simulink model "sampleModel106"  (R2022a)
settings: Solver=VariableStepAuto  StartTime=0.0  StopTime=10.0  RelTol=1e-3
undefined symbols (not defined in the file): DiscIntNeverNeededParam, magnitude, Newton, Raphson
libraries: simulink x379, slpidlib x89
(part 3 of 16)

== system sampleModel106/cfblk74/cfblk13/cfblk11 ==
  cfblk1 : Inport
  cfblk12 : Inport  Port=2
  cfblk10 : Subsystem
  cfblk11 : If  IfExpression=u1 >= 0  SampleTime=1
  cfblk14 : Subsystem  TreatAsAtomicUnit=on
  cfblk15 : Subsystem  TreatAsAtomicUnit=on
  cfblk{16..20} (5 alike) : Delay  SampleTime=1
  cfblk3 : slpidlib/PID Controller (2DOF)  Controller=PID  Form=Parallel  TimeDomain=Discrete-time  UseExternalTs=off  SampleTime=1  IntegratorMethod=Forward Euler  FilterMethod=Forward Euler  ControllerParametersSource=internal  P=1  I=1  UseKiTs=off  D=0  N=100  UseFilter=on  b=1  c=1  TunerSelectOption=Transfer Function Based (PID Tuner App)  InitialConditionSource=internal  InitialConditionForIntegrator=0  InitialConditionForFilter=0  DifferentiatorICPrevScaledInput=0  ExternalReset=none  TrackingMode=off  Kt=1  LimitOutput=off  SatLimitsSource=internal  UpperSaturationLimit=inf  LowerSaturationLimit=-inf  LinearizeAsGain=off  AntiWindupMode=none  Kb=1  POutMin=[]  POutMax=[]  IOutMin=[]  IOutMax=[]  DOutMin=[]  DOutMax=[]  NOutMin=[]  NOutMax=[]  bOutMin=[]  bOutMax=[]  cOutMin=[]  cOutMax=[]  SumOutMin=[]  SumOutMax=[]  SaturationOutMin=[]  SaturationOutMax=[]  PParamMin=[]  PParamMax=[]  IParamMin=[]  IParamMax=[]  DParamMin=[]  DParamMax=[]  NParamMin=[]  NParamMax=[]  bParamMin=[]  bParamMax=[]  cParamMin=[]  cParamMax=[]  KbParamMin=[]  KbParamMax=[]  KtParamMin=[]  KtParamMax=[]  KbOutMin=[]  KbOutMax=[]  KtOutMin=[]  KtOutMax=[]  IntegratorOutMin=[]  IntegratorOutMax=[]  FilterOutMin=[]  FilterOutMax=[]  SumI1OutMin=[]  SumI1OutMax=[]  SumI2OutMin=[]  SumI2OutMax=[]  SumI3OutMin=[]  SumI3OutMax=[]  SumI4OutMin=[]  SumI4OutMax=[]  SumDOutMin=[]  SumDOutMax=[]  Sum1OutMin=[]  Sum1OutMax=[]  Sum2OutMin=[]  Sum2OutMax=[]  Sum3OutMin=[]  Sum3OutMax=[]  DifferentiatorOutMin=[]  DifferentiatorOutMax=[]  FilterDiffOutCoefMin=[]  FilterDiffOutCoefMax=[]  ReciprocalOutMin=[]  ReciprocalOutMax=[]  SumDenOutMin=[]  SumDenOutMax=[]  SumNumOutMin=[]  SumNumOutMax=[]  DivideOutMin=[]  DivideOutMax=[]  UdiffTsProdOutMin=[]  UdiffTsProdOutMax=[]  NTsProdOutMin=[]  NTsProdOutMax=[]  UintegralTsProdOutMin=[]  UintegralTsProdOutMax=[]  UngainTsProdOutMin=[]  UngainTsProdOutMax=[]  IntegratorContinuousStateAttributes=''  IntegratorStateMustResolveToSignalObject=off  IntegratorRTWStateStorageClass=Auto  FilterContinuousStateAttributes=''  FilterStateMustResolveToSignalObject=off  FilterRTWStateStorageClass=Auto  ParallelPVariant=InternalParameters  IdealPVariant=Disabled  IVariant=InternalParameters  DVariant=InternalParameters  bVariant=InternalParameters  cVariant=InternalParameters  IntegratorVariant=Discrete  SatVariant=Disabled  AWVariant=Passthrough  PCopyVariant=Disabled  TRVariant=Disabled  FdbkBlocksVariant=Forward  IdealPFdbkVariant=Disabled  SatFdbkVariant=Disabled  DerivativeFilterVariant=ForwardEulerFilter  NVariant=InternalParameters  NCopyVariant=Disabled  FilterICVariant=InternalICsFilter  IntegratorICVariant=InternalICs  ExternalResetVariant=Disabled  TRSumVariant=Passthrough  SumFdbkVariant=Disabled  SumVariant=Sum_PID  TsampFilterVariant=InternalTs  TsampNgainVariant=Passthrough  TsampIntegralVariant=Passthrough  ExternalSaturationOutDataTypeStr=Inherit: Same as second input
      settings: SourceProductBaseCode=SL
  cfblk4 : DiscreteFilter  SampleTime=1
  cfblk5 : Squeeze
  cfblk6 : Constant  Value=[-862764176.620188]  SampleTime=1
  cfblk7 : Subsystem
  cfblk8 : Subsystem
  cfblk9 : Subsystem
  cfblk2 : Outport
  cfblk13 : Outport  Port=2
  wires:
  cfblk4/1 -> cfblk5/1, cfblk3/2, cfblk15/4(cfblk9)
  cfblk9/1(cfblk2) -> cfblk4/1
  cfblk1/1 -> cfblk10/1(cfblk1), cfblk15/5(cfblk10), cfblk15/6(cfblk11)
  cfblk3/1 -> cfblk13/1
  cfblk10/1(cfblk2) -> cfblk2/1
  cfblk14/2(cfblk15) -> cfblk8/1(cfblk1)
  cfblk9/2(cfblk11) -> cfblk7/1(cfblk1)
  cfblk12/1 -> cfblk7/2(cfblk11)
  cfblk9/3(cfblk12) -> cfblk14/1(cfblk1), cfblk7/6(cfblk15)
  cfblk6/1 -> cfblk14/2(cfblk13)
  cfblk10/2(cfblk11) -> cfblk9/3(cfblk10)
  cfblk10/3(cfblk12) -> cfblk14/3(cfblk14)
  cfblk14/4(cfblk17) -> cfblk8/2(cfblk13), cfblk15/1(cfblk1)
  cfblk15/1(cfblk2) -> cfblk7/3(cfblk12)
  cfblk10/4(cfblk13) -> cfblk8/3(cfblk14)
  cfblk5/1 -> cfblk7/4(cfblk13), cfblk15/3(cfblk8)
  cfblk10/5(cfblk14) -> cfblk11/1
  cfblk8/1(cfblk2) -> cfblk7/5(cfblk14)
  cfblk8/2(cfblk15) -> cfblk3/1, cfblk19/1
  cfblk11/1 -> cfblk14/Action
  cfblk11/2 -> cfblk15/Action
  cfblk7/1(cfblk2) -> cfblk16/1
  cfblk16/1 -> cfblk10/2(cfblk9)
  cfblk7/2(cfblk16) -> cfblk17/1
  cfblk17/1 -> cfblk9/2(cfblk9)
  cfblk14/1(cfblk2) -> cfblk18/1
  cfblk18/1 -> cfblk9/1(cfblk1)
  cfblk19/1 -> cfblk15/2(cfblk7)
  cfblk14/3(cfblk16) -> cfblk20/1
  cfblk20/1 -> cfblk10/3(cfblk10)

== system sampleModel106/cfblk74/cfblk13/cfblk12 ==
  cfblk1 : Inport
  cfblk11 : Inport  Port=2
  cfblk12 : Inport  Port=3
  cfblk13 : Inport  Port=4
  cfblk10 : Subsystem
  cfblk3 : simulink/Discrete/Transfer Fcn First Order  PoleZ=0.95  ICPrevOutput=0.0  DoSatur=off
  cfblk4 : DiscreteTransferFcn  SampleTime=1
  cfblk5 : simulink/Discrete/Difference  ICPrevInput=0.0  OutMin=[]  OutMax=[]  OutDataTypeStr=Inherit: Inherit via back propagation  OutDataType=fixdt(1, 16)  OutScaling=2^-10  DoSatur=off
  cfblk6 : Math  Operator=mod
  cfblk7 : Product  Inputs=**
  cfblk8 : Constant  Value=[-371034601.961383]  SampleTime=1
  cfblk9 : Constant  Value=[478763481.548670]  SampleTime=1
  cfblk2 : Outport
  cfblk14 : Outport  Port=2
  wires:
  cfblk1/1 -> cfblk7/1
  cfblk13/1 -> cfblk4/1
  cfblk9/1 -> cfblk5/1
  cfblk10/1(cfblk2) -> cfblk6/1
  cfblk4/1 -> cfblk10/1(cfblk1)
  cfblk10/2(cfblk10) -> cfblk6/2
  cfblk3/1 -> cfblk7/2
  cfblk8/1 -> cfblk10/2(cfblk8)
  cfblk11/1 -> cfblk14/1
  cfblk6/1 -> cfblk2/1
  cfblk5/1 -> cfblk3/1
  cfblk12/1 -> cfblk10/3(cfblk9)

== system sampleModel106/cfblk74/cfblk13/cfblk13 ==
  cfblk1 : Inport
  cfblk13 : Inport  Port=2
  cfblk14 : Inport  Port=3
  cfblk10 : Subsystem
  cfblk11 : Subsystem
  cfblk12 : Subsystem
  cfblk15 : Delay  SampleTime=1
  cfblk16 : Delay  SampleTime=1
  cfblk3 : Delay  DelayLengthSource=Input port  SampleTime=1
      settings: InputPortMap=u0,p1
  cfblk4 : Product  Inputs=*
  cfblk5 : MinMax  Function=max  Inputs=3
  cfblk6 : Constant  Value=[-504496130.229108]  SampleTime=1
  cfblk7 : Constant  Value=[-450280739.885704]  SampleTime=1
  cfblk8 : Constant  Value=[-820475792.542349]  SampleTime=1
  cfblk9 : Subsystem
  cfblk2 : Outport
  wires:
  cfblk13/1 -> cfblk4/1
  cfblk14/1 -> cfblk12/1(cfblk1), cfblk10/5(cfblk15)
  cfblk11/1(cfblk2) -> cfblk10/1(cfblk1)
  cfblk4/1 -> cfblk11/1(cfblk1)
  cfblk5/1 -> cfblk3/1
  cfblk7/1 -> cfblk5/2
  cfblk9/1(cfblk2) -> cfblk5/3
  cfblk6/1 -> cfblk2/1
  cfblk8/1 -> cfblk10/2(cfblk12)
  cfblk12/1(cfblk2) -> cfblk3/2
  cfblk1/1 -> cfblk10/4(cfblk14)
  cfblk12/2(cfblk12) -> cfblk9/1(cfblk1)
  cfblk10/1(cfblk2) -> cfblk9/2(cfblk7)
  cfblk3/1 -> cfblk15/1
  cfblk15/1 -> cfblk5/1
  cfblk9/2(cfblk8) -> cfblk16/1
  cfblk16/1 -> cfblk10/3(cfblk13)

== system sampleModel106/cfblk74/cfblk9/cfblk10 ==
  cfblk1 : Inport
  cfblk7 : Inport  Port=2
  cfblk3 : DiscreteZeroPole  Poles=[0 0.5]  Gain=1
  cfblk4 : Reshape
  cfblk5 : Sum  Inputs=+
  cfblk6 : Constant  Value=[-238352155.093476]  SampleTime=1
  cfblk2 : Outport
  wires:
  cfblk6/1 -> cfblk3/1
  cfblk5/1 -> cfblk4/1
  cfblk4/1 -> cfblk2/1
  cfblk7/1 -> cfblk5/1

== system sampleModel106/cfblk74/cfblk9/cfblk11 ==
  cfblk1 : Inport
  cfblk10 : Inport  Port=2
  cfblk11 : Delay  SampleTime=1
  cfblk12 : Delay  SampleTime=1
  cfblk3 : slpidlib/PID Controller (2DOF)  Controller=PID  Form=Parallel  TimeDomain=Discrete-time  UseExternalTs=off  SampleTime=1  IntegratorMethod=Forward Euler  FilterMethod=Forward Euler  ControllerParametersSource=internal  P=1  I=1  UseKiTs=off  D=0  N=100  UseFilter=on  b=1  c=1  TunerSelectOption=Transfer Function Based (PID Tuner App)  InitialConditionSource=internal  InitialConditionForIntegrator=0  InitialConditionForFilter=0  DifferentiatorICPrevScaledInput=0  ExternalReset=none  TrackingMode=off  Kt=1  LimitOutput=off  SatLimitsSource=internal  UpperSaturationLimit=inf  LowerSaturationLimit=-inf  LinearizeAsGain=off  AntiWindupMode=none  Kb=1  POutMin=[]  POutMax=[]  IOutMin=[]  IOutMax=[]  DOutMin=[]  DOutMax=[]  NOutMin=[]  NOutMax=[]  bOutMin=[]  bOutMax=[]  cOutMin=[]  cOutMax=[]  SumOutMin=[]  SumOutMax=[]  SaturationOutMin=[]  SaturationOutMax=[]  PParamMin=[]  PParamMax=[]  IParamMin=[]  IParamMax=[]  DParamMin=[]  DParamMax=[]  NParamMin=[]  NParamMax=[]  bParamMin=[]  bParamMax=[]  cParamMin=[]  cParamMax=[]  KbParamMin=[]  KbParamMax=[]  KtParamMin=[]  KtParamMax=[]  KbOutMin=[]  KbOutMax=[]  KtOutMin=[]  KtOutMax=[]  IntegratorOutMin=[]  IntegratorOutMax=[]  FilterOutMin=[]  FilterOutMax=[]  SumI1OutMin=[]  SumI1OutMax=[]  SumI2OutMin=[]  SumI2OutMax=[]  SumI3OutMin=[]  SumI3OutMax=[]  SumI4OutMin=[]  SumI4OutMax=[]  SumDOutMin=[]  SumDOutMax=[]  Sum1OutMin=[]  Sum1OutMax=[]  Sum2OutMin=[]  Sum2OutMax=[]  Sum3OutMin=[]  Sum3OutMax=[]  DifferentiatorOutMin=[]  DifferentiatorOutMax=[]  FilterDiffOutCoefMin=[]  FilterDiffOutCoefMax=[]  ReciprocalOutMin=[]  ReciprocalOutMax=[]  SumDenOutMin=[]  SumDenOutMax=[]  SumNumOutMin=[]  SumNumOutMax=[]  DivideOutMin=[]  DivideOutMax=[]  UdiffTsProdOutMin=[]  UdiffTsProdOutMax=[]  NTsProdOutMin=[]  NTsProdOutMax=[]  UintegralTsProdOutMin=[]  UintegralTsProdOutMax=[]  UngainTsProdOutMin=[]  UngainTsProdOutMax=[]  IntegratorContinuousStateAttributes=''  IntegratorStateMustResolveToSignalObject=off  IntegratorRTWStateStorageClass=Auto  FilterContinuousStateAttributes=''  FilterStateMustResolveToSignalObject=off  FilterRTWStateStorageClass=Auto  ParallelPVariant=InternalParameters  IdealPVariant=Disabled  IVariant=InternalParameters  DVariant=InternalParameters  bVariant=InternalParameters  cVariant=InternalParameters  IntegratorVariant=Discrete  SatVariant=Disabled  AWVariant=Passthrough  PCopyVariant=Disabled  TRVariant=Disabled  FdbkBlocksVariant=Forward  IdealPFdbkVariant=Disabled  SatFdbkVariant=Disabled  DerivativeFilterVariant=ForwardEulerFilter  NVariant=InternalParameters  NCopyVariant=Disabled  FilterICVariant=InternalICsFilter  IntegratorICVariant=InternalICs  ExternalResetVariant=Disabled  TRSumVariant=Passthrough  SumFdbkVariant=Disabled  SumVariant=Sum_PID  TsampFilterVariant=InternalTs  TsampNgainVariant=Passthrough  TsampIntegralVariant=Passthrough  ExternalSaturationOutDataTypeStr=Inherit: Same as second input
      settings: SourceProductBaseCode=SL
  cfblk4 : DiscreteTransferFcn  SampleTime=1
  cfblk5 : DotProduct  OutDataTypeStr=Inherit: Inherit via internal rule
  cfblk6 : ComplexToMagnitudeAngle
  cfblk7 : Constant  Value=[-659082313.129839]  SampleTime=1
  cfblk8 : Subsystem
  cfblk9 : Subsystem
  cfblk2 : Outport
  wires:
  cfblk9/1(cfblk2) -> cfblk4/1
  cfblk10/1 -> cfblk9/1(cfblk1)
  cfblk3/1 -> cfblk6/1
  cfblk7/1 -> cfblk8/2(cfblk9)
  cfblk8/1(cfblk2) -> cfblk2/1
  cfblk6/1 -> cfblk8/3(cfblk10)
  cfblk1/1 -> cfblk3/2
  cfblk8/2(cfblk11) -> cfblk9/2(cfblk8)
  cfblk4/1 -> cfblk5/1
  cfblk6/2 -> cfblk5/2
  cfblk5/1 -> cfblk11/1
  cfblk11/1 -> cfblk8/1(cfblk1)
  cfblk9/2(cfblk9) -> cfblk12/1
  cfblk12/1 -> cfblk3/1

== system sampleModel106/cfblk74/cfblk9/cfblk12 ==
  cfblk1 : Inport
  cfblk10 : Subsystem
  cfblk11 : If  IfExpression=u1 >= 0  SampleTime=1
  cfblk13 : Subsystem  TreatAsAtomicUnit=on
  cfblk14 : Subsystem  TreatAsAtomicUnit=on
  cfblk{15..21} (7 alike) : Delay  SampleTime=1
  cfblk3 : UnaryMinus
  cfblk4 : Sum  Inputs=+-
  cfblk5 : Squeeze
  cfblk6 : Constant  Value=[744843425.057498]  SampleTime=1
  cfblk7 : Constant  Value=[784568269.900237]  SampleTime=1
  cfblk8 : Subsystem
  cfblk9 : Subsystem
  cfblk2 : Outport
  cfblk12 : Outport  Port=2
  wires:
  cfblk1/1 -> cfblk8/1(cfblk1), cfblk9/2(cfblk8)
  cfblk5/1 -> cfblk12/1, cfblk9/4(cfblk10), cfblk2/1
  cfblk9/1(cfblk2) -> cfblk14/2(cfblk9)
  cfblk6/1 -> cfblk13/1(cfblk1), cfblk4/1, cfblk4/2
  cfblk7/1 -> cfblk10/1(cfblk1), cfblk9/3(cfblk9)
  cfblk4/1 -> cfblk14/3(cfblk10)
  cfblk8/1(cfblk2) -> cfblk5/1
  cfblk14/1(cfblk2) -> cfblk10/3(cfblk7)
  cfblk10/1(cfblk2) -> cfblk15/1, cfblk20/1, cfblk21/1
  cfblk14/2(cfblk12) -> cfblk13/2(cfblk12)
  cfblk13/4(cfblk16) -> cfblk3/1
  cfblk11/1 -> cfblk13/Action
  cfblk11/2 -> cfblk14/Action
  cfblk15/1 -> cfblk14/4(cfblk11)
  cfblk13/1(cfblk2) -> cfblk16/1
  cfblk16/1 -> cfblk10/2(cfblk6)
  cfblk13/2(cfblk14) -> cfblk17/1
  cfblk17/1 -> cfblk8/2(cfblk7)
  cfblk13/3(cfblk15) -> cfblk18/1
  cfblk18/1 -> cfblk9/1(cfblk1)
  cfblk3/1 -> cfblk19/1
  cfblk19/1 -> cfblk14/1(cfblk1)
  cfblk20/1 -> cfblk11/1
  cfblk21/1 -> cfblk13/3(cfblk13)

== system sampleModel106/cfblk74/cfblk9/cfblk13 ==
  cfblk1 : Inport
  cfblk10 : Delay  SampleTime=1
  cfblk3 : Sum  Inputs=|++
  cfblk4 : Constant  Value=[-872842553.263368]  SampleTime=1
  cfblk5 : Subsystem
  cfblk6 : Subsystem
  cfblk7 : Subsystem
  cfblk8 : Delay  SampleTime=1
  cfblk9 : Delay  SampleTime=1
  cfblk2 : Outport
  wires:
  cfblk5/1(cfblk2) -> cfblk3/1
  cfblk3/1 -> cfblk7/1(cfblk1)
  cfblk1/1 -> cfblk6/1(cfblk1)
  cfblk4/1 -> cfblk3/2
  cfblk5/2(cfblk10) -> cfblk9/1, cfblk10/1
  cfblk6/1(cfblk2) -> cfblk5/2(cfblk9)
  cfblk7/2(cfblk13) -> cfblk2/1
  cfblk7/1(cfblk2) -> cfblk8/1
  cfblk8/1 -> cfblk5/1(cfblk1)
  cfblk9/1 -> cfblk6/2(cfblk7)
  cfblk10/1 -> cfblk6/3(cfblk8)

== system sampleModel106/cfblk74/cfblk9/cfblk14 ==
  cfblk1 : Inport
  cfblk7 : Inport  Port=2
  cfblk3 : DiscreteIntegrator  ICPrevOutput=DiscIntNeverNeededParam  ICPrevScaledInput=DiscIntNeverNeededParam
  cfblk4 : DiscreteTransferFcn  SampleTime=1
  cfblk5 : PermuteDimensions
  cfblk6 : ComplexToRealImag
  cfblk2 : Outport
  cfblk8 : Outport  Port=2
  cfblk9 : Outport  Port=3
  cfblk10 : Outport  Port=4
  wires:
  cfblk7/1 -> cfblk10/1, cfblk5/1
  cfblk6/1 -> cfblk9/1
  cfblk5/1 -> cfblk3/1
  cfblk6/2 -> cfblk4/1
  cfblk4/1 -> cfblk2/1
  cfblk1/1 -> cfblk8/1
  cfblk3/1 -> cfblk6/1

== system sampleModel106/cfblk74/cfblk9/cfblk15 ==
  cfblk1 : Inport
  cfblk12 : Inport  Port=2
  cfblk10 : Subsystem
  cfblk11 : Subsystem
  cfblk{3,13..16} (5 alike) : Delay  SampleTime=1
  cfblk4 : Sum  Inputs=--
  cfblk5 : Trigonometry
  cfblk6 : Reshape
  cfblk7 : Rounding
  cfblk8 : Constant  Value=[-157824095.994580]  SampleTime=1
  cfblk9 : Subsystem
  cfblk2 : Outport
  wires:
  cfblk5/1 -> cfblk3/1
  cfblk9/1(cfblk2) -> cfblk5/1
  cfblk3/1 -> cfblk7/1
  cfblk7/1 -> cfblk14/1, cfblk15/1
  cfblk8/1 -> cfblk2/1
  cfblk1/1 -> cfblk4/1
  cfblk4/1 -> cfblk11/2(cfblk13)
  cfblk12/1 -> cfblk10/1(cfblk1)
  cfblk6/1 -> cfblk10/2(cfblk11)
  cfblk10/1(cfblk2) -> cfblk9/1(cfblk1)
  cfblk11/2(cfblk15) -> cfblk9/2(cfblk7)
  cfblk11/3(cfblk16) -> cfblk9/3(cfblk8)
  cfblk11/1(cfblk2) -> cfblk13/1
  cfblk13/1 -> cfblk4/2
  cfblk14/1 -> cfblk11/1(cfblk1)
  cfblk15/1 -> cfblk11/3(cfblk14)
  cfblk10/2(cfblk12) -> cfblk16/1
  cfblk16/1 -> cfblk6/1

== system sampleModel106/cfblk74/cfblk9/cfblk16 ==
  cfblk1 : Inport
  cfblk10 : Delay  SampleTime=1
  cfblk3 : simulink/Discrete/Transfer Fcn Lead or Lag  PoleZ=0.95  ZeroZ=0.75  ICPrevOutput=0.0  ICPrevInput=0.0  DoSatur=off
      settings: SourceProductBaseCode=SL
  cfblk4 : simulink/Discrete/Difference  ICPrevInput=0.0  OutMin=[]  OutMax=[]  OutDataTypeStr=Inherit: Inherit via back propagation  OutDataType=fixdt(1, 16)  OutScaling=2^-10  DoSatur=off
  cfblk5 : Math  Operator=hypot
  cfblk6 : Constant  Value=[599464047.475240]  SampleTime=1
  cfblk7 : Subsystem
  cfblk8 : Subsystem
  cfblk2 : Outport
  cfblk9 : Outport  Port=2
  wires:
  cfblk6/1 -> cfblk8/1(cfblk1), cfblk8/3(cfblk15)
  cfblk8/1(cfblk2) -> cfblk5/1
  cfblk4/1 -> cfblk5/2, cfblk8/2(cfblk14)
  cfblk7/1(cfblk2) -> cfblk4/1
  cfblk1/1 -> cfblk3/1, cfblk7/3(cfblk8)
  cfblk8/2(cfblk16) -> cfblk2/1
  cfblk3/1 -> cfblk7/2(cfblk7), cfblk9/1
  cfblk5/1 -> cfblk10/1
  cfblk10/1 -> cfblk7/1(cfblk1)

== system sampleModel106/cfblk74/cfblk9/cfblk9 ==
  cfblk1 : Inport
  cfblk12 : Inport  Port=2
  cfblk10 : Subsystem
  cfblk11 : Subsystem
  cfblk13 : Delay  SampleTime=1
  cfblk3 : Sqrt  Operator=rSqrt  AlgorithmType=Newton-Raphson
  cfblk4 : Abs  SaturateOnIntegerOverflow=off
  cfblk5 : simulink/Math Operations/Slider Gain  gain=1  low=0  high=2
  cfblk6 : Constant  Value=[-816000564.261839]  SampleTime=1
  cfblk7 : Constant  Value=[352712742.183147]  SampleTime=1
  cfblk8 : Constant  Value=[982731264.482814]  SampleTime=1
  cfblk9 : Subsystem
  cfblk2 : Outport
  wires:
  cfblk11/1(cfblk2) -> cfblk9/1(cfblk1)
  cfblk1/1 -> cfblk11/1(cfblk1)
  cfblk12/1 -> cfblk5/1
  cfblk7/1 -> cfblk11/2(cfblk6), cfblk10/4(cfblk12)
  cfblk4/1 -> cfblk2/1
  cfblk3/1 -> cfblk4/1
  cfblk9/1(cfblk2) -> cfblk10/1(cfblk1)
  cfblk6/1 -> cfblk3/1
  cfblk9/2(cfblk11) -> cfblk10/2(cfblk10)
  cfblk8/1 -> cfblk11/4(cfblk8)
  cfblk5/1 -> cfblk10/3(cfblk11)
  cfblk10/1(cfblk2) -> cfblk13/1
  cfblk13/1 -> cfblk11/3(cfblk7)

== system sampleModel106/cfblk75/cfblk5/cfblk10 ==
  cfblk1 : Inport
  cfblk10 : Subsystem  TreatAsAtomicUnit=on
  cfblk11 : Subsystem  TreatAsAtomicUnit=on
  cfblk{12..15} (4 alike) : Delay  SampleTime=1
  cfblk3 : UnitDelay  HasFrameUpgradeWarning=on
  cfblk4 : Assignment  DiagnosticForDimensions=Warning  IndexOptions=Index vector (dialog)  Indices=1  OutputSizes=1
  cfblk5 : Product
  cfblk6 : Constant  Value=[-997108857.142024]  SampleTime=1
  cfblk7 : Subsystem
  cfblk8 : Subsystem
  cfblk9 : If  IfExpression=u1 >= 0  SampleTime=1
  cfblk2 : Outport
  wires:
  cfblk8/1(cfblk2) -> cfblk3/1
  cfblk4/1 -> cfblk11/2(cfblk6), cfblk13/1
  cfblk7/1(cfblk2) -> cfblk5/1
  cfblk10/1(cfblk2) -> cfblk14/1, cfblk15/1
  cfblk5/1 -> cfblk8/1(cfblk1), cfblk8/2(cfblk9), cfblk11/1(cfblk1), cfblk12/1
  cfblk6/1 -> cfblk2/1
  cfblk7/2(cfblk10) -> cfblk4/1, cfblk10/2(cfblk7)
  cfblk11/1(cfblk2) -> cfblk10/1(cfblk1)
  cfblk1/1 -> cfblk7/3(cfblk9)
  cfblk3/1 -> cfblk4/2, cfblk11/3(cfblk7)
  cfblk9/1 -> cfblk10/Action
  cfblk9/2 -> cfblk11/Action
  cfblk12/1 -> cfblk7/2(cfblk8)
  cfblk13/1 -> cfblk7/1(cfblk1)
  cfblk14/1 -> cfblk5/2
  cfblk15/1 -> cfblk9/1

== system sampleModel106/cfblk75/cfblk5/cfblk11 ==
  cfblk1 : Inport
  cfblk11 : Inport  Port=2
  cfblk12 : Inport  Port=3
  cfblk13 : Inport  Port=4
  cfblk10 : Subsystem
  cfblk3 : UnitDelay  HasFrameUpgradeWarning=on
  cfblk4 : DiscreteZeroPole  Poles=[0 0.5]  Gain=1
  cfblk5 : PermuteDimensions
  cfblk6 : Reshape
  cfblk7 : Reshape
  cfblk8 : Constant  Value=[-896470513.555038]  SampleTime=1
  cfblk9 : Constant  Value=[798275808.792166]  SampleTime=1
  cfblk2 : Outport
  wires:
  cfblk11/1 -> cfblk5/1
  cfblk12/1 -> cfblk4/1
  cfblk7/1 -> cfblk2/1
  cfblk13/1 -> cfblk6/1
  cfblk5/1 -> cfblk7/1
  cfblk8/1 -> cfblk3/1
  cfblk4/1 -> cfblk10/1(cfblk1)
  cfblk6/1 -> cfblk10/2(cfblk9)
  cfblk1/1 -> cfblk10/3(cfblk10)

== system sampleModel106/cfblk75/cfblk5/cfblk9 ==
  cfblk1 : Inport
  cfblk10 : Subsystem
  cfblk12 : Delay  SampleTime=1
  cfblk13 : Delay  SampleTime=1
  cfblk14 : Delay  SampleTime=1
  cfblk3 : Signum
  cfblk4 : simulink/Math Operations/MinMax Running Resettable  Function=min  vinit=0.0
  cfblk5 : Product  Inputs=**
  cfblk6 : Math  Operator=pow
  cfblk7 : Constant  Value=[881073384.469198]  SampleTime=1
  cfblk8 : Subsystem
  cfblk9 : Subsystem
  cfblk2 : Outport
  cfblk11 : Outport  Port=2
  wires:
  cfblk6/1 -> cfblk10/1(cfblk1), cfblk10/3(cfblk15)
  cfblk9/1(cfblk2) -> cfblk2/1, cfblk4/2
  cfblk7/1 -> cfblk9/1(cfblk1), cfblk8/2(cfblk8)
  cfblk4/1 -> cfblk5/1, cfblk14/1
  cfblk1/1 -> cfblk11/1, cfblk8/1(cfblk1), cfblk4/1
  cfblk5/1 -> cfblk3/1
  cfblk8/1(cfblk2) -> cfblk6/1, cfblk5/2
  cfblk3/1 -> cfblk12/1, cfblk13/1
  cfblk10/1(cfblk2) -> cfblk9/2(cfblk16)
  cfblk12/1 -> cfblk6/2
  cfblk13/1 -> cfblk8/3(cfblk9)
  cfblk14/1 -> cfblk10/2(cfblk14)

== system sampleModel106/cfblk75/cfblk6/cfblk5 ==
  cfblk1 : Inport
  cfblk8 : Inport  Port=2
  cfblk9 : Inport  Port=3
  cfblk10 : Inport  Port=4
  cfblk3 : UnitDelay  HasFrameUpgradeWarning=on
  cfblk4 : Reshape
  cfblk5 : Sum  Inputs=-+
  cfblk6 : Abs  SaturateOnIntegerOverflow=off
  cfblk7 : Subsystem
  cfblk2 : Outport
  wires:
  cfblk3/1 -> cfblk4/1
  cfblk1/1 -> cfblk2/1
  cfblk10/1 -> cfblk6/1
  cfblk7/1(cfblk2) -> cfblk5/1
  cfblk5/1 -> cfblk3/1
  cfblk9/1 -> cfblk7/1(cfblk1)
  cfblk8/1 -> cfblk7/2(cfblk9)
  cfblk6/1 -> cfblk5/2

== system sampleModel106/cfblk75/cfblk6/cfblk6 ==
  cfblk1 : Inport
  cfblk15 : Inport  Port=2
  cfblk16 : Inport  Port=3
  cfblk17 : Inport  Port=4
  cfblk10 : Polyval  Coefs=[ +2.081618890e-019, -1.441693666e-014, +4.719686976e-010, -8.536869453e-006, +1.621573104e-001, -8.087801117e+001 ]
  cfblk11 : Sin  TimeSource=Use external signal  SampleTime=0
  cfblk12 : ComplexToMagnitudeAngle
  cfblk13 : Subsystem
  cfblk14 : Subsystem
  cfblk18 : Delay  SampleTime=1
  cfblk3 : simulink/Discrete/Transfer Fcn Real Zero  ZeroZ=0.75  ICPrevInput=0.0  DoSatur=off
      settings: SourceProductBaseCode=SL
  cfblk4 : slpidlib/PID Controller  Controller=PID  Form=Parallel  TimeDomain=Discrete-time  UseExternalTs=off  SampleTime=1  IntegratorMethod=Forward Euler  FilterMethod=Forward Euler  ControllerParametersSource=internal  P=1  I=1  UseKiTs=off  D=0  N=100  UseFilter=on  TunerSelectOption=Transfer Function Based (PID Tuner App)  InitialConditionSource=internal  InitialConditionForIntegrator=0  InitialConditionForFilter=0  DifferentiatorICPrevScaledInput=0  ExternalReset=none  TrackingMode=off  Kt=1  LimitOutput=off  SatLimitsSource=internal  UpperSaturationLimit=inf  LowerSaturationLimit=-inf  LinearizeAsGain=off  AntiWindupMode=none  Kb=1  POutMin=[]  POutMax=[]  IOutMin=[]  IOutMax=[]  DOutMin=[]  DOutMax=[]  NOutMin=[]  NOutMax=[]  SumOutMin=[]  SumOutMax=[]  SaturationOutMin=[]  SaturationOutMax=[]  PParamMin=[]  PParamMax=[]  IParamMin=[]  IParamMax=[]  DParamMin=[]  DParamMax=[]  NParamMin=[]  NParamMax=[]  KbParamMin=[]  KbParamMax=[]  KtParamMin=[]  KtParamMax=[]  KbOutMin=[]  KbOutMax=[]  KtOutMin=[]  KtOutMax=[]  IntegratorOutMin=[]  IntegratorOutMax=[]  FilterOutMin=[]  FilterOutMax=[]  SumI1OutMin=[]  SumI1OutMax=[]  SumI2OutMin=[]  SumI2OutMax=[]  SumI3OutMin=[]  SumI3OutMax=[]  SumI4OutMin=[]  SumI4OutMax=[]  SumDOutMin=[]  SumDOutMax=[]  DifferentiatorOutMin=[]  DifferentiatorOutMax=[]  FilterDiffOutCoefMin=[]  FilterDiffOutCoefMax=[]  ReciprocalOutMin=[]  ReciprocalOutMax=[]  SumDenOutMin=[]  SumDenOutMax=[]  SumNumOutMin=[]  SumNumOutMax=[]  DivideOutMin=[]  DivideOutMax=[]  UdiffTsProdOutMin=[]  UdiffTsProdOutMax=[]  NTsProdOutMin=[]  NTsProdOutMax=[]  UintegralTsProdOutMin=[]  UintegralTsProdOutMax=[]  UngainTsProdOutMin=[]  UngainTsProdOutMax=[]  IntegratorContinuousStateAttributes=''  IntegratorStateMustResolveToSignalObject=off  IntegratorRTWStateStorageClass=Auto  FilterContinuousStateAttributes=''  FilterStateMustResolveToSignalObject=off  FilterRTWStateStorageClass=Auto  ParallelPVariant=InternalParameters  IdealPVariant=Disabled  IVariant=InternalParameters  DVariant=InternalParameters  IntegratorVariant=Discrete  SatVariant=Disabled  AWVariant=Passthrough  PCopyVariant=Disabled  TRVariant=Disabled  FdbkBlocksVariant=Forward  IdealPFdbkVariant=Disabled  SatFdbkVariant=Disabled  DerivativeFilterVariant=ForwardEulerFilter  NVariant=InternalParameters  NCopyVariant=Disabled  FilterICVariant=InternalICsFilter  IntegratorICVariant=InternalICs  ExternalResetVariant=Disabled  TRSumVariant=Passthrough  SumFdbkVariant=Disabled  SumVariant=Sum_PID  TsampFilterVariant=InternalTs  TsampNgainVariant=Passthrough  TsampIntegralVariant=Passthrough  ExternalSaturationOutDataTypeStr=Inherit: Same as second input  aMode=0
  cfblk5 : DiscreteTransferFcn  SampleTime=1
  cfblk6 : ComplexToMagnitudeAngle
  cfblk7 : simulink/Math Operations/Slider Gain  gain=1  low=0  high=2
  cfblk8 : Product  Inputs=**
  cfblk9 : ComplexToMagnitudeAngle
  cfblk2 : Outport
  wires:
  cfblk16/1 -> cfblk13/1(cfblk1)
  cfblk3/1 -> cfblk8/1
  cfblk5/1 -> cfblk14/1(cfblk1)
  cfblk10/1 -> cfblk5/1
  cfblk17/1 -> cfblk10/1
  cfblk15/1 -> cfblk12/1
  cfblk6/1 -> cfblk11/1
  cfblk1/1 -> cfblk9/1
  cfblk4/1 -> cfblk2/1
  cfblk8/1 -> cfblk6/1
  cfblk6/2 -> cfblk7/1
  cfblk7/1 -> cfblk4/1
  cfblk12/1 -> cfblk14/2(cfblk12)
  cfblk14/1(cfblk2) -> cfblk13/2(cfblk9)
  cfblk12/2 -> cfblk8/2
  cfblk11/1 -> cfblk14/3(cfblk13)
  cfblk13/1(cfblk2) -> cfblk18/1
  cfblk18/1 -> cfblk3/1

== system sampleModel106/cfblk75/cfblk6/cfblk7 ==
  cfblk1 : Inport
  cfblk10 : Inport  Port=2
  cfblk11 : Delay  SampleTime=1
  cfblk3 : DiscreteFilter  SampleTime=1
  cfblk4 : PermuteDimensions
  cfblk5 : MinMax  Function=max  Inputs=2
  cfblk6 : Sqrt  Operator=rSqrt  AlgorithmType=Newton-Raphson
  cfblk7 : Constant  Value=[196330297.271654]  SampleTime=1
  cfblk8 : Constant  Value=[327342414.725762]  SampleTime=1
  cfblk9 : Subsystem
  cfblk2 : Outport
  wires:
  cfblk8/1 -> cfblk2/1, cfblk9/3(cfblk9)
  cfblk7/1 -> cfblk3/1
  cfblk1/1 -> cfblk5/2
  cfblk10/1 -> cfblk9/1(cfblk1)
  cfblk4/1 -> cfblk6/1
  cfblk3/1 -> cfblk9/2(cfblk8)
  cfblk5/1 -> cfblk4/1, cfblk9/4(cfblk10)
  cfblk6/1 -> cfblk11/1
  cfblk11/1 -> cfblk5/1

== system sampleModel106/cfblk75/cfblk6/cfblk8 ==
  cfblk1 : Inport
  cfblk13 : Inport  Port=2
  cfblk14 : Inport  Port=3
  cfblk10 : Subsystem
  cfblk11 : Subsystem
  cfblk12 : Subsystem
  cfblk16 : Delay  SampleTime=1
  cfblk3 : Math
  cfblk4 : DotProduct  OutDataTypeStr=Inherit: Inherit via internal rule
  cfblk5 : Sin  TimeSource=Use external signal  SampleTime=0
  cfblk6 : Reshape
  cfblk7 : Constant  Value=[-655048019.730096]  SampleTime=1
  cfblk8 : Constant  Value=[-645308090.557076]  SampleTime=1
  cfblk9 : Subsystem
  cfblk2 : Outport
  cfblk15 : Outport  Port=2
  wires:
  cfblk13/1 -> cfblk10/1(cfblk1)
  cfblk9/1(cfblk2) -> cfblk10/2(cfblk10)
  cfblk3/1 -> cfblk10/3(cfblk11)
  cfblk14/1 -> cfblk11/1(cfblk1)
  cfblk10/1(cfblk2) -> cfblk15/1
  cfblk6/1 -> cfblk10/4(cfblk12)
  cfblk12/1(cfblk2) -> cfblk6/1
  cfblk1/1 -> cfblk9/1(cfblk1)
  cfblk7/1 -> cfblk9/2(cfblk11)
  cfblk8/1 -> cfblk2/1
  cfblk9/2(cfblk13) -> cfblk5/1
  cfblk5/1 -> cfblk11/2(cfblk10)
  cfblk9/3(cfblk14) -> cfblk4/1
  cfblk11/1(cfblk2) -> cfblk12/1(cfblk1)
  cfblk9/4(cfblk15) -> cfblk3/1, cfblk4/2
  cfblk11/2(cfblk11) -> cfblk12/2(cfblk8)
  cfblk4/1 -> cfblk16/1
  cfblk16/1 -> cfblk9/3(cfblk12)

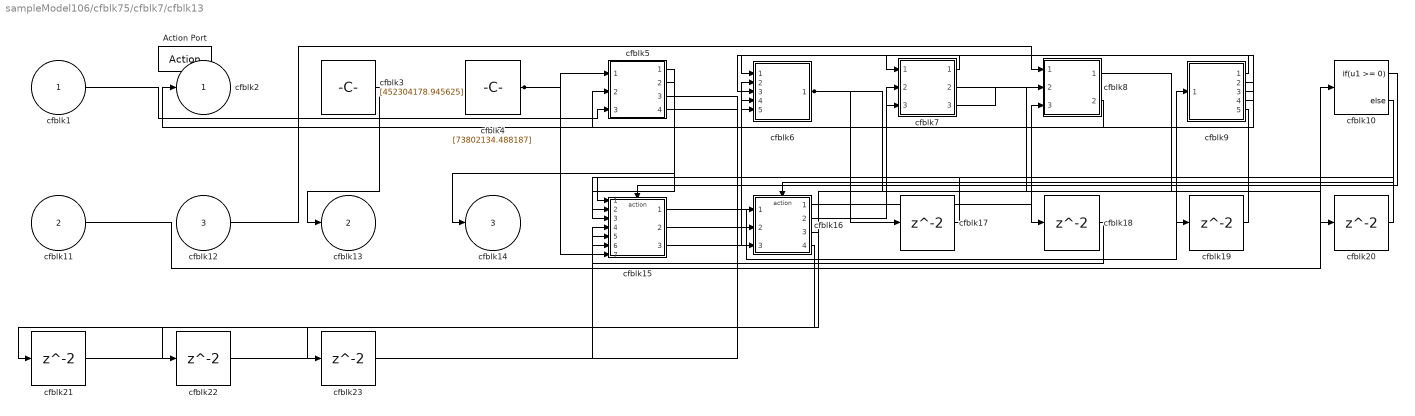
== system sampleModel106/cfblk75/cfblk7/cfblk13 ==
  cfblk1 : Inport
  cfblk11 : Inport  Port=2
  cfblk12 : Inport  Port=3
  Action Port : ActionPort  ActionPortLabel=if(u1 >= 0)
  cfblk10 : If  IfExpression=u1 >= 0  SampleTime=1
  cfblk15 : Subsystem  TreatAsAtomicUnit=on
  cfblk16 : Subsystem  TreatAsAtomicUnit=on
  cfblk{17..23} (7 alike) : Delay
  cfblk3 : Constant  Value=[452304178.945625]  SampleTime=1
  cfblk4 : Constant  Value=[73802134.488187]  SampleTime=1
  cfblk5 : Subsystem
  cfblk6 : Subsystem
  cfblk7 : Subsystem
  cfblk8 : Subsystem
  cfblk9 : Subsystem
  cfblk2 : Outport
  cfblk13 : Outport  Port=2
  cfblk14 : Outport  Port=3
  wires:
  cfblk7/1(cfblk2) -> cfblk6/1(cfblk1)
  cfblk3/1 -> cfblk13/1
  cfblk4/1 -> cfblk5/1(cfblk1), cfblk15/7(cfblk11)
  cfblk15/1(cfblk2) -> cfblk9/1(cfblk1)
  cfblk12/1 -> cfblk8/1(cfblk1)
  cfblk6/1(cfblk2) -> cfblk17/1, cfblk18/1
  cfblk5/1(cfblk2) -> cfblk14/1
  cfblk15/2(cfblk12) -> cfblk6/2(cfblk8)
  cfblk9/1(cfblk2) -> cfblk6/3(cfblk9)
  cfblk9/2(cfblk14) -> cfblk6/4(cfblk10)
  cfblk8/2(cfblk11) -> cfblk2/1
  cfblk11/1 -> cfblk10/1
  cfblk15/3(cfblk13) -> cfblk6/5(cfblk11)
  cfblk7/3(cfblk12) -> cfblk8/2(cfblk9)
  cfblk1/1 -> cfblk5/3(cfblk12)
  cfblk16/1(cfblk2) -> cfblk8/3(cfblk10)
  cfblk9/3(cfblk15) -> cfblk7/1(cfblk1)
  cfblk16/2(cfblk14) -> cfblk7/2(cfblk9)
  cfblk5/2(cfblk13) -> cfblk15/3(cfblk7)
  cfblk9/4(cfblk16) -> cfblk7/3(cfblk10)
  cfblk5/3(cfblk14) -> cfblk16/1(cfblk1)
  cfblk5/4(cfblk15) -> cfblk16/3(cfblk13)
  cfblk10/1 -> cfblk15/Action
  cfblk10/2 -> cfblk16/Action
  cfblk17/1 -> cfblk15/2(cfblk6)
  cfblk18/1 -> cfblk15/6(cfblk10)
  cfblk7/2(cfblk11) -> cfblk19/1
  cfblk19/1 -> cfblk5/2(cfblk11)
  cfblk8/1(cfblk2) -> cfblk20/1
  cfblk20/1 -> cfblk15/1(cfblk1)
  cfblk9/5(cfblk17) -> cfblk21/1
  cfblk21/1 -> cfblk16/2(cfblk12)
  cfblk16/3(cfblk15) -> cfblk22/1
  cfblk22/1 -> cfblk15/4(cfblk8)
  cfblk16/4(cfblk16) -> cfblk23/1
  cfblk23/1 -> cfblk15/5(cfblk9)

== system sampleModel106/cfblk75/cfblk7/cfblk14 ==
  cfblk1 : Inport
  Action Port : ActionPort  ActionPortLabel=else
  cfblk10 : Subsystem
  cfblk11 : Delay
  cfblk12 : Delay
  cfblk3 : simulink/Discrete/Difference  ICPrevInput=0.0  OutMin=[]  OutMax=[]  OutDataTypeStr=Inherit: Inherit via back propagation  OutDataType=fixdt(1, 16)  OutScaling=2^-10  DoSatur=off
  cfblk4 : Squeeze
  cfblk5 : Constant  Value=[-923686366.439134]  SampleTime=1
  cfblk6 : Subsystem
  cfblk7 : Subsystem
  cfblk8 : Subsystem
  cfblk9 : Subsystem
  cfblk2 : Outport
  wires:
  cfblk6/1(cfblk2) -> cfblk7/1(cfblk1), cfblk8/5(cfblk11)
  cfblk3/1 -> cfblk10/1(cfblk1)
  cfblk4/1 -> cfblk9/1(cfblk1)
  cfblk9/1(cfblk2) -> cfblk10/2(cfblk9), cfblk8/3(cfblk9)
  cfblk5/1 -> cfblk4/1
  cfblk8/1(cfblk2) -> cfblk2/1
  cfblk1/1 -> cfblk8/1(cfblk1)
  cfblk10/1(cfblk2) -> cfblk6/2(cfblk7)
  cfblk10/2(cfblk10) -> cfblk8/2(cfblk8)
  cfblk10/3(cfblk11) -> cfblk8/4(cfblk10), cfblk12/1
  cfblk7/1(cfblk2) -> cfblk11/1
  cfblk11/1 -> cfblk6/1(cfblk1)
  cfblk12/1 -> cfblk3/1

== system sampleModel106/cfblk75/cfblk7/cfblk8 ==
  cfblk1 : Inport
  cfblk11 : Inport  Port=2
  cfblk10 : Subsystem
  cfblk13 : Delay  SampleTime=1
  cfblk14 : Delay  SampleTime=1
  cfblk15 : Delay  SampleTime=1
  cfblk3 : DiscreteTransferFcn  SampleTime=1
  cfblk4 : Signum
  cfblk5 : Assignment  DiagnosticForDimensions=Warning  IndexOptions=Index vector (dialog)  Indices=1  OutputSizes=1
  cfblk6 : ComplexToMagnitudeAngle
  cfblk7 : Constant  Value=[488066147.040023]  SampleTime=1
  cfblk8 : Constant  Value=[103352949.139322]  SampleTime=1
  cfblk9 : Subsystem
  cfblk2 : Outport
  cfblk12 : Outport  Port=2
  wires:
  cfblk4/1 -> cfblk9/1(cfblk1)
  cfblk1/1 -> cfblk5/2
  cfblk8/1 -> cfblk12/1
  cfblk7/1 -> cfblk10/1(cfblk1)
  cfblk10/1(cfblk2) -> cfblk6/1
  cfblk5/1 -> cfblk3/1
  cfblk11/1 -> cfblk10/2(cfblk8)
  cfblk10/3(cfblk11) -> cfblk2/1
  cfblk9/1(cfblk2) -> cfblk10/3(cfblk9)
  cfblk3/1 -> cfblk13/1
  cfblk13/1 -> cfblk5/1
  cfblk6/1 -> cfblk14/1
  cfblk14/1 -> cfblk4/1
  cfblk10/2(cfblk10) -> cfblk15/1
  cfblk15/1 -> cfblk9/2(cfblk7)

== system sampleModel106/cfblk75/cfblk7/cfblk9 ==
  cfblk1 : Inport
  cfblk8 : Inport  Port=2
  cfblk10 : Delay  SampleTime=1
  cfblk11 : Delay  SampleTime=1
  cfblk3 : DiscreteFir  SampleTime=1
  cfblk4 : Polyval  Coefs=[ +2.081618890e-019, -1.441693666e-014, +4.719686976e-010, -8.536869453e-006, +1.621573104e-001, -8.087801117e+001 ]
  cfblk5 : Constant  Value=[383424715.224345]  SampleTime=1
  cfblk6 : Subsystem
  cfblk7 : Subsystem
  cfblk2 : Outport
  cfblk9 : Outport  Port=2
  wires:
  cfblk8/1 -> cfblk2/1
  cfblk5/1 -> cfblk4/1
  cfblk6/1(cfblk2) -> cfblk9/1, cfblk7/2(cfblk14)
  cfblk7/2(cfblk15) -> cfblk3/1
  cfblk1/1 -> cfblk6/2(cfblk12)
  cfblk4/1 -> cfblk7/1(cfblk1)
  cfblk7/1(cfblk2) -> cfblk10/1
  cfblk10/1 -> cfblk6/1(cfblk1)
  cfblk3/1 -> cfblk11/1
  cfblk11/1 -> cfblk6/3(cfblk13)

== system sampleModel106/cfblk76/cfblk4/cfblk10 ==
  cfblk1 : Inport
  cfblk10 : Inport  Port=2
  cfblk11 : Delay  SampleTime=1
  cfblk12 : Delay  SampleTime=1
  cfblk13 : Delay  SampleTime=1
  cfblk3 : DiscreteFir  SampleTime=1
  cfblk4 : Rounding
  cfblk5 : Sum  Inputs=+
  cfblk6 : Product
  cfblk7 : Assignment  DiagnosticForDimensions=Warning  IndexOptions=Index vector (dialog)  Indices=1  OutputSizes=1
  cfblk8 : Subsystem
  cfblk9 : Subsystem
  cfblk2 : Outport
  wires:
  cfblk6/1 -> cfblk8/1(cfblk1)
  cfblk1/1 -> cfblk3/1
  cfblk9/1(cfblk2) -> cfblk5/1
  cfblk3/1 -> cfblk7/1
  cfblk7/1 -> cfblk2/1, cfblk6/2
  cfblk8/2(cfblk7) -> cfblk4/1, cfblk9/2(cfblk8)
  cfblk10/1 -> cfblk8/2(cfblk6)
  cfblk8/1(cfblk2) -> cfblk11/1
  cfblk11/1 -> cfblk6/1
  cfblk4/1 -> cfblk12/1
  cfblk12/1 -> cfblk7/2
  cfblk5/1 -> cfblk13/1
  cfblk13/1 -> cfblk9/1(cfblk1)

== system sampleModel106/cfblk76/cfblk4/cfblk9 ==
  cfblk1 : Inport
  cfblk6 : Inport  Port=2
  cfblk7 : Inport  Port=3
  cfblk8 : Inport  Port=4
  cfblk10 : Subsystem  TreatAsAtomicUnit=on
  cfblk11 : Delay  SampleTime=1
  cfblk12 : Delay  SampleTime=1
  cfblk13 : Delay  SampleTime=1
  cfblk3 : Subsystem
  cfblk4 : Subsystem
  cfblk5 : If  IfExpression=u1 >= 0  SampleTime=1
  cfblk9 : Subsystem  TreatAsAtomicUnit=on
  cfblk2 : Outport
  wires:
  cfblk8/1 -> cfblk2/1
  cfblk6/1 -> cfblk5/1
  cfblk7/1 -> cfblk10/1(cfblk1)
  cfblk1/1 -> cfblk10/2(cfblk7)
  cfblk3/1(cfblk2) -> cfblk4/1(cfblk1)
  cfblk10/1(cfblk2) -> cfblk3/3(cfblk9)
  cfblk5/1 -> cfblk9/Action
  cfblk5/2 -> cfblk10/Action
  cfblk4/1(cfblk2) -> cfblk11/1
  cfblk11/1 -> cfblk9/1(cfblk1)
  cfblk9/1(cfblk2) -> cfblk12/1
  cfblk12/1 -> cfblk3/1(cfblk1)
  cfblk4/2(cfblk8) -> cfblk13/1
  cfblk13/1 -> cfblk3/2(cfblk8)

== system sampleModel106/cfblk76/cfblk5/cfblk6 ==
  cfblk1 : Inport
  cfblk10 : Inport  Port=2
  cfblk12 : Delay  SampleTime=1
  cfblk13 : Delay  SampleTime=1
  cfblk14 : Delay  SampleTime=1
  cfblk3 : DiscreteTransferFcn  SampleTime=1
  cfblk4 : DiscreteZeroPole  Poles=[0 0.5]  Gain=1
  cfblk5 : Sum  Inputs=+-
  cfblk6 : Constant  Value=[-371925363.409586]  SampleTime=1
  cfblk7 : Constant  Value=[575701262.165620]  SampleTime=1
  cfblk8 : Subsystem
  cfblk9 : Subsystem
  cfblk2 : Outport
  cfblk11 : Outport  Port=2
  wires:
  cfblk10/1 -> cfblk9/1(cfblk1)
  cfblk6/1 -> cfblk2/1
  cfblk7/1 -> cfblk9/2(cfblk10)
  cfblk5/1 -> cfblk8/2(cfblk8)
  cfblk8/1(cfblk2) -> cfblk11/1
  cfblk8/2(cfblk11) -> cfblk9/3(cfblk11)
  cfblk9/1(cfblk2) -> cfblk4/1
  cfblk1/1 -> cfblk3/1, cfblk8/4(cfblk10)
  cfblk3/1 -> cfblk5/1
  cfblk4/1 -> cfblk12/1
  cfblk12/1 -> cfblk8/1(cfblk1)
  cfblk9/2(cfblk12) -> cfblk13/1
  cfblk13/1 -> cfblk8/3(cfblk9)
  cfblk8/3(cfblk12) -> cfblk14/1
  cfblk14/1 -> cfblk5/2

== system sampleModel106/cfblk76/cfblk7/cfblk8 ==
  cfblk1 : Inport
  cfblk10 : Constant  Value=[-568952145.099277]  SampleTime=1
  cfblk11 : Subsystem
  cfblk12 : Subsystem
  cfblk13 : Subsystem
  cfblk14 : Subsystem
  cfblk15 : Subsystem
  cfblk16 : Subsystem
  cfblk17 : Delay  SampleTime=1
  cfblk18 : Delay  SampleTime=1
  cfblk3 : simulink/Discrete/Transfer Fcn First Order  PoleZ=0.95  ICPrevOutput=0.0  DoSatur=off
  cfblk4 : Delay  DelayLengthSource=Input port  SampleTime=1
      settings: InputPortMap=u0,p1
  cfblk5 : Product
  cfblk6 : MinMax  Inputs=3
  cfblk7 : Polyval  Coefs=[ +2.081618890e-019, -1.441693666e-014, +4.719686976e-010, -8.536869453e-006, +1.621573104e-001, -8.087801117e+001 ]
  cfblk8 : PermuteDimensions
  cfblk9 : Gain  Gain=[-769317553.596711]
  cfblk2 : Outport
  wires:
  cfblk12/1(cfblk2) -> cfblk14/1(cfblk1)
  cfblk16/1(cfblk2) -> cfblk12/1(cfblk1)
  cfblk1/1 -> cfblk4/1, cfblk15/5(cfblk11)
  cfblk11/1(cfblk2) -> cfblk15/1(cfblk1)
  cfblk9/1 -> cfblk15/2(cfblk8), cfblk6/1
  cfblk8/1 -> cfblk5/1
  cfblk14/1(cfblk2) -> cfblk7/1
  cfblk3/1 -> cfblk12/2(cfblk10), cfblk15/3(cfblk9), cfblk12/4(cfblk12), cfblk6/2
  cfblk7/1 -> cfblk13/1(cfblk1)
  cfblk12/2(cfblk13) -> cfblk9/1, cfblk15/4(cfblk10)
  cfblk6/1 -> cfblk2/1
  cfblk15/2(cfblk12) -> cfblk8/1
  cfblk10/1 -> cfblk11/1(cfblk1), cfblk11/3(cfblk15), cfblk3/1
  cfblk4/1 -> cfblk16/1(cfblk1)
  cfblk14/2(cfblk12) -> cfblk13/2(cfblk11)
  cfblk13/1(cfblk2) -> cfblk11/2(cfblk14)
  cfblk13/2(cfblk12) -> cfblk5/2, cfblk6/3
  cfblk15/1(cfblk2) -> cfblk17/1
  cfblk17/1 -> cfblk4/2
  cfblk5/1 -> cfblk18/1
  cfblk18/1 -> cfblk12/3(cfblk11)

== system sampleModel106/cfblk77/cfblk11/cfblk5 ==
  cfblk1 : Inport
  cfblk10 : Subsystem  TreatAsAtomicUnit=on
  cfblk11 : Subsystem  TreatAsAtomicUnit=on
  cfblk{12..18} (7 alike) : Delay
  cfblk3 : Product  Inputs=*
  cfblk4 : Constant  Value=[-833827322.265856]  SampleTime=1
  cfblk5 : Constant  Value=[-765577698.877952]  SampleTime=1
  cfblk6 : Subsystem
  cfblk7 : Subsystem
  cfblk8 : Subsystem
  cfblk9 : If  IfExpression=u1 >= 0  SampleTime=1
  cfblk2 : Outport
  wires:
  cfblk8/1(cfblk2) -> cfblk7/1(cfblk1)
  cfblk8/2(cfblk11) -> cfblk7/2(cfblk7), cfblk15/1, cfblk16/1, cfblk17/1
  cfblk10/1(cfblk2) -> cfblk2/1
  cfblk5/1 -> cfblk3/1
  cfblk11/3(cfblk12) -> cfblk8/1(cfblk1)
  cfblk10/3(cfblk13) -> cfblk8/2(cfblk9)
  cfblk4/1 -> cfblk6/3(cfblk5)
  cfblk3/1 -> cfblk8/3(cfblk10), cfblk10/3(cfblk8)
  cfblk1/1 -> cfblk6/4(cfblk6), cfblk10/2(cfblk7)
  cfblk6/1(cfblk2) -> cfblk11/2(cfblk10)
  cfblk6/2(cfblk7) -> cfblk10/1(cfblk1)
  cfblk9/1 -> cfblk10/Action
  cfblk9/2 -> cfblk11/Action
  cfblk11/1(cfblk2) -> cfblk12/1
  cfblk12/1 -> cfblk6/1(cfblk1)
  cfblk10/2(cfblk12) -> cfblk13/1
  cfblk13/1 -> cfblk6/2(cfblk4)
  cfblk7/1(cfblk2) -> cfblk14/1
  cfblk14/1 -> cfblk11/1(cfblk1)
  cfblk15/1 -> cfblk10/4(cfblk9)
  cfblk16/1 -> cfblk10/5(cfblk10)
  cfblk17/1 -> cfblk10/6(cfblk11)
  cfblk11/2(cfblk11) -> cfblk18/1
  cfblk18/1 -> cfblk9/1

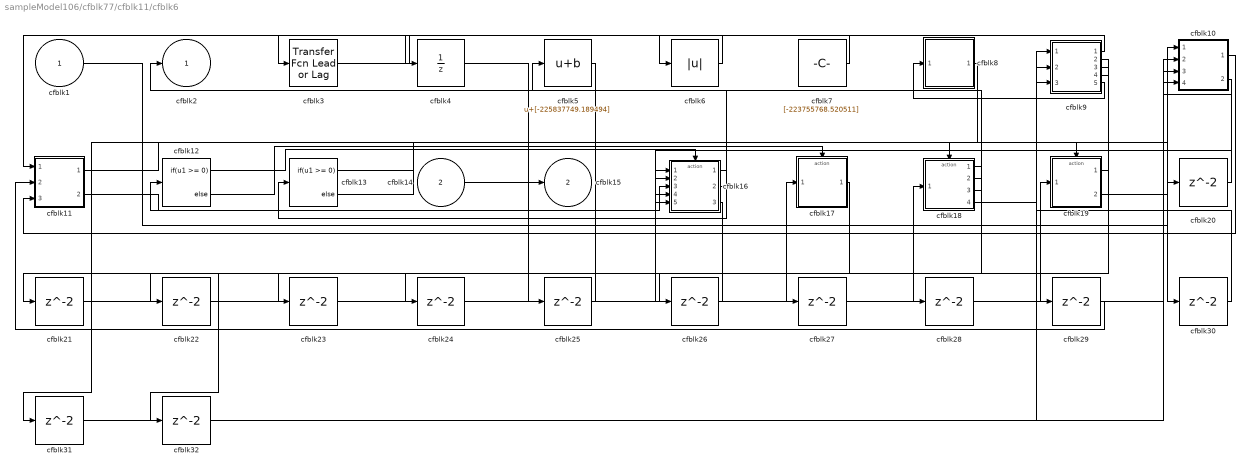
== system sampleModel106/cfblk77/cfblk11/cfblk6 ==
  cfblk1 : Inport
  cfblk14 : Inport  Port=2
  cfblk10 : Subsystem
  cfblk11 : Subsystem
  cfblk12 : If  IfExpression=u1 >= 0  SampleTime=1
  cfblk13 : If  IfExpression=u1 >= 0  SampleTime=1
  cfblk16 : Subsystem  TreatAsAtomicUnit=on
  cfblk17 : Subsystem  TreatAsAtomicUnit=on
  cfblk18 : Subsystem  TreatAsAtomicUnit=on
  cfblk19 : Subsystem  TreatAsAtomicUnit=on
  cfblk{20..32} (13 alike) : Delay
  cfblk3 : simulink/Discrete/Transfer Fcn Lead or Lag  PoleZ=0.95  ZeroZ=0.75  ICPrevOutput=0.0  ICPrevInput=0.0  DoSatur=off
      settings: SourceProductBaseCode=SL
  cfblk4 : UnitDelay  SampleTime=-1  HasFrameUpgradeWarning=on
  cfblk5 : Bias  Bias=[-225837749.189494]  SaturateOnIntegerOverflow=off
  cfblk6 : Abs  SaturateOnIntegerOverflow=off
  cfblk7 : Constant  Value=[-223755768.520511]  SampleTime=1
  cfblk8 : Subsystem
  cfblk9 : Subsystem
  cfblk2 : Outport
  cfblk15 : Outport  Port=2
  wires:
  cfblk7/1 -> cfblk11/1(cfblk1)
  cfblk9/1(cfblk2) -> cfblk3/1
  cfblk3/1 -> cfblk6/1
  cfblk16/1(cfblk2) -> cfblk13/1
  cfblk1/1 -> cfblk10/1(cfblk1)
  cfblk16/2(cfblk13) -> cfblk2/1
  cfblk18/2(cfblk13) -> cfblk5/1
  cfblk6/1 -> cfblk4/1
  cfblk14/1 -> cfblk15/1
  cfblk11/2(cfblk16) -> cfblk16/3(cfblk10)
  cfblk9/5(cfblk12) -> cfblk8/1(cfblk1)
  cfblk18/4(cfblk15) -> cfblk9/3(cfblk8)
  cfblk10/1(cfblk2) -> cfblk11/3(cfblk15)
  cfblk10/2(cfblk11) -> cfblk16/5(cfblk12)
  cfblk12/1 -> cfblk16/Action
  cfblk12/2 -> cfblk17/Action
  cfblk13/1 -> cfblk18/Action
  cfblk13/2 -> cfblk19/Action
  cfblk11/1(cfblk2) -> cfblk20/1
  cfblk20/1 -> cfblk10/3(cfblk9)
  cfblk18/1(cfblk2) -> cfblk21/1
  cfblk21/1 -> cfblk17/1(cfblk1)
  cfblk17/1(cfblk2) -> cfblk22/1
  cfblk22/1 -> cfblk18/1(cfblk1)
  cfblk5/1 -> cfblk23/1
  cfblk23/1 -> cfblk16/1(cfblk1)
  cfblk18/3(cfblk14) -> cfblk24/1
  cfblk24/1 -> cfblk16/4(cfblk11)
  cfblk4/1 -> cfblk25/1
  cfblk25/1 -> cfblk12/1
  cfblk9/2(cfblk9) -> cfblk26/1
  cfblk26/1 -> cfblk16/2(cfblk9)
  cfblk9/3(cfblk10) -> cfblk27/1
  cfblk27/1 -> cfblk10/2(cfblk8)
  cfblk9/4(cfblk11) -> cfblk28/1
  cfblk28/1 -> cfblk19/1(cfblk1)
  cfblk19/1(cfblk2) -> cfblk29/1
  cfblk29/1 -> cfblk11/2(cfblk14)
  cfblk19/2(cfblk7) -> cfblk30/1
  cfblk30/1 -> cfblk9/2(cfblk7)
  cfblk8/1(cfblk2) -> cfblk31/1
  cfblk31/1 -> cfblk9/1(cfblk1)
  cfblk16/3(cfblk14) -> cfblk32/1
  cfblk32/1 -> cfblk10/4(cfblk10)

== system sampleModel106/cfblk77/cfblk12/cfblk6 ==
  cfblk1 : Inport
  cfblk{9..13} (5 alike) : Delay
  cfblk3 : DiscreteIntegrator  SampleTime=-1  ICPrevOutput=DiscIntNeverNeededParam  ICPrevScaledInput=DiscIntNeverNeededParam
  cfblk4 : Sum  Inputs=+-
  cfblk5 : Subsystem
  cfblk6 : Subsystem
  cfblk7 : Subsystem
  cfblk8 : Subsystem
  cfblk2 : Outport
  wires:
  cfblk3/1 -> cfblk4/1
  cfblk7/1(cfblk2) -> cfblk5/1(cfblk1)
  cfblk5/1(cfblk2) -> cfblk6/1(cfblk1)
  cfblk7/2(cfblk12) -> cfblk8/1(cfblk1), cfblk5/2(cfblk11), cfblk2/1
  cfblk8/1(cfblk2) -> cfblk4/2
  cfblk8/2(cfblk10) -> cfblk3/1, cfblk13/1
  cfblk1/1 -> cfblk7/1(cfblk1)
  cfblk4/1 -> cfblk9/1, cfblk10/1, cfblk11/1, cfblk12/1
  cfblk6/1(cfblk2) -> cfblk8/2(cfblk9)
  cfblk9/1 -> cfblk7/2(cfblk11)
  cfblk10/1 -> cfblk6/2(cfblk10)
  cfblk11/1 -> cfblk5/4(cfblk13)
  cfblk12/1 -> cfblk5/5(cfblk14)
  cfblk13/1 -> cfblk5/3(cfblk12)

== system sampleModel106/cfblk78/cfblk11/cfblk6 ==
  cfblk1 : Inport
  cfblk16 : Inport  Port=2
  cfblk17 : Inport  Port=3
  cfblk10 : Constant  Value=[606580708.738063]  SampleTime=1
  cfblk11 : Constant  Value=[-379418196.415275]  SampleTime=1
  cfblk12 : Constant  Value=[-559971844.060398]  SampleTime=1
  cfblk13 : Subsystem
  cfblk14 : Subsystem
  cfblk15 : Subsystem
  cfblk{18..21} (4 alike) : Delay
  cfblk3 : DiscreteZeroPole  Poles=[0 0.5]  Gain=1  SampleTime=-1
  cfblk4 : Delay  ShowEnablePort=on
      settings: InputPortMap=u0,e6
  cfblk5 : Assignment  DiagnosticForDimensions=Warning  IndexOptions=Index vector (dialog)  Indices=1  OutputSizes=1
  cfblk6 : Sum  Inputs=+-
  cfblk7 : Squeeze
  cfblk8 : Math  Operator=pow
  cfblk9 : MinMax  Inputs=2
  cfblk2 : Outport
  wires:
  cfblk1/1 -> cfblk5/1
  cfblk16/1 -> cfblk15/1(cfblk1)
  cfblk3/1 -> cfblk8/1
  cfblk5/1 -> cfblk3/1
  cfblk15/1(cfblk2) -> cfblk14/1(cfblk1)
  cfblk6/1 -> cfblk4/1
  cfblk14/2(cfblk15) -> cfblk4/2
  cfblk14/3(cfblk16) -> cfblk2/1
  cfblk15/2(cfblk16) -> cfblk14/2(cfblk13)
  cfblk11/1 -> cfblk7/1
  cfblk12/1 -> cfblk9/1
  cfblk13/1(cfblk2) -> cfblk9/2
  cfblk7/1 -> cfblk13/1(cfblk1)
  cfblk14/4(cfblk17) -> cfblk13/2(cfblk12), cfblk6/2
  cfblk10/1 -> cfblk13/3(cfblk13), cfblk6/1
  cfblk15/3(cfblk17) -> cfblk14/3(cfblk14)
  cfblk17/1 -> cfblk8/2
  cfblk8/1 -> cfblk15/5(cfblk15)
  cfblk14/1(cfblk2) -> cfblk18/1
  cfblk18/1 -> cfblk5/2
  cfblk4/1 -> cfblk19/1
  cfblk19/1 -> cfblk15/2(cfblk12)
  cfblk9/1 -> cfblk20/1
  cfblk20/1 -> cfblk15/3(cfblk13)
  cfblk13/2(cfblk14) -> cfblk21/1
  cfblk21/1 -> cfblk15/4(cfblk14)

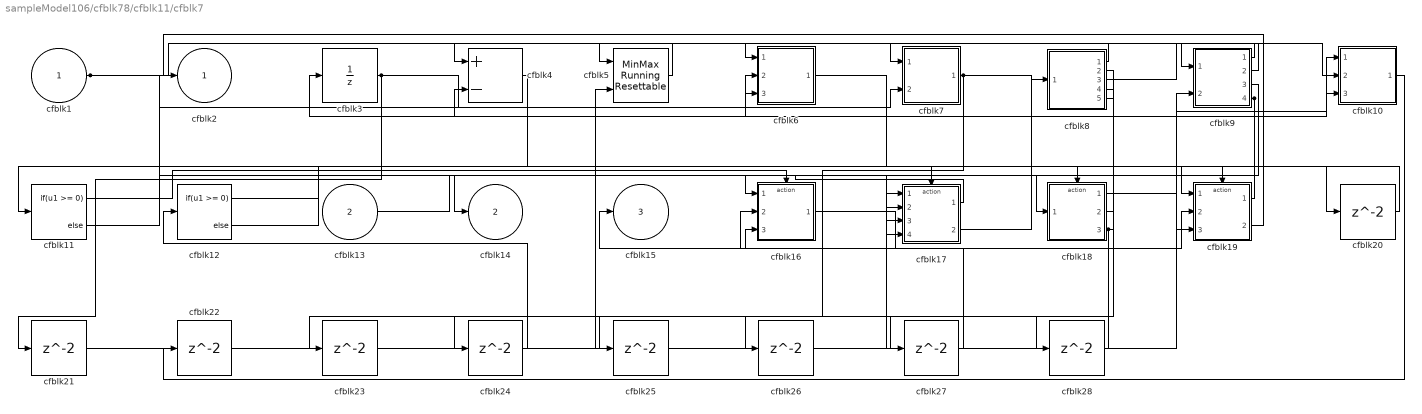
== system sampleModel106/cfblk78/cfblk11/cfblk7 ==
  cfblk1 : Inport
  cfblk13 : Inport  Port=2
  cfblk10 : Subsystem
  cfblk11 : If  IfExpression=u1 >= 0  SampleTime=1
  cfblk12 : If  IfExpression=u1 >= 0  SampleTime=1
  cfblk16 : Subsystem  TreatAsAtomicUnit=on
  cfblk17 : Subsystem  TreatAsAtomicUnit=on
  cfblk18 : Subsystem  TreatAsAtomicUnit=on
  cfblk19 : Subsystem  TreatAsAtomicUnit=on
  cfblk{20..28} (9 alike) : Delay
  cfblk3 : UnitDelay  SampleTime=-1  HasFrameUpgradeWarning=on
  cfblk4 : Sum  Inputs=+-
  cfblk5 : simulink/Math Operations/MinMax Running Resettable  Function=min  vinit=0.0
  cfblk6 : Subsystem
  cfblk7 : Subsystem
  cfblk8 : Subsystem
  cfblk9 : Subsystem
  cfblk2 : Outport
  cfblk14 : Outport  Port=2
  cfblk15 : Outport  Port=3
  wires:
  cfblk1/1 -> cfblk9/1(cfblk1), cfblk19/3(cfblk13), cfblk7/2(cfblk8)
  cfblk9/1(cfblk2) -> cfblk5/1
  cfblk9/2(cfblk6) -> cfblk6/1(cfblk1)
  cfblk16/1(cfblk2) -> cfblk19/2(cfblk12)
  cfblk17/1(cfblk2) -> cfblk14/1
  cfblk4/1 -> cfblk11/1
  cfblk19/1(cfblk2) -> cfblk3/1
  cfblk19/2(cfblk14) -> cfblk2/1
  cfblk13/1 -> cfblk18/1(cfblk1)
  cfblk8/1(cfblk2) -> cfblk7/1(cfblk1)
  cfblk18/1(cfblk2) -> cfblk10/1(cfblk1)
  cfblk5/1 -> cfblk4/1
  cfblk7/1(cfblk2) -> cfblk10/3(cfblk12), cfblk24/1, cfblk25/1
  cfblk17/2(cfblk13) -> cfblk8/1(cfblk1)
  cfblk3/1 -> cfblk6/2(cfblk8), cfblk21/1
  cfblk8/3(cfblk15) -> cfblk10/2(cfblk11)
  cfblk9/3(cfblk7) -> cfblk16/1(cfblk1)
  cfblk9/4(cfblk8) -> cfblk4/2, cfblk17/4(cfblk12)
  cfblk18/3(cfblk7) -> cfblk15/1, cfblk6/3(cfblk9)
  cfblk11/1 -> cfblk16/Action
  cfblk11/2 -> cfblk17/Action
  cfblk12/1 -> cfblk18/Action
  cfblk12/2 -> cfblk19/Action
  cfblk6/1(cfblk2) -> cfblk20/1
  cfblk20/1 -> cfblk19/1(cfblk1)
  cfblk21/1 -> cfblk17/2(cfblk10)
  cfblk10/1(cfblk2) -> cfblk22/1
  cfblk22/1 -> cfblk17/1(cfblk1)
  cfblk18/2(cfblk6) -> cfblk23/1
  cfblk23/1 -> cfblk5/2
  cfblk24/1 -> cfblk12/1
  cfblk25/1 -> cfblk17/3(cfblk11)
  cfblk8/2(cfblk14) -> cfblk26/1
  cfblk26/1 -> cfblk9/2(cfblk5)
  cfblk8/4(cfblk16) -> cfblk27/1
  cfblk27/1 -> cfblk16/2(cfblk12)
  cfblk8/5(cfblk17) -> cfblk28/1
  cfblk28/1 -> cfblk16/3(cfblk13)

== system sampleModel106/cfblk78/cfblk12/cfblk4 ==
  cfblk1 : Inport
  cfblk11 : Inport  Port=2
  cfblk12 : Inport  Port=3
  cfblk13 : Inport  Port=4
  cfblk10 : If  IfExpression=u1 >= 0  SampleTime=1
  cfblk16 : Subsystem  TreatAsAtomicUnit=on
  cfblk17 : Subsystem  TreatAsAtomicUnit=on
  cfblk18 : Delay
  cfblk19 : Delay
  cfblk20 : Delay
  cfblk3 : Delay  DelayLengthSource=Input port
      settings: InputPortMap=u0,p1
  cfblk4 : ComplexToMagnitudeAngle
  cfblk5 : Math  Operator=log
  cfblk6 : Sum  Inputs=+
  cfblk7 : Constant  Value=[-314971435.165244]  SampleTime=1
  cfblk8 : Subsystem
  cfblk9 : Subsystem
  cfblk2 : Outport
  cfblk14 : Outport  Port=2
  cfblk15 : Outport  Port=3
  wires:
  cfblk17/1(cfblk2) -> cfblk9/1(cfblk1)
  cfblk16/1(cfblk2) -> cfblk15/1
  cfblk12/1 -> cfblk4/1
  cfblk16/2(cfblk13) -> cfblk5/1
  cfblk17/2(cfblk8) -> cfblk9/2(cfblk8)
  cfblk9/1(cfblk2) -> cfblk2/1
  cfblk7/1 -> cfblk10/1
  cfblk6/1 -> cfblk3/1
  cfblk17/3(cfblk9) -> cfblk16/2(cfblk11)
  cfblk11/1 -> cfblk6/1
  cfblk9/2(cfblk9) -> cfblk8/1(cfblk1)
  cfblk8/1(cfblk2) -> cfblk18/1, cfblk19/1
  cfblk13/1 -> cfblk3/2
  cfblk4/1 -> cfblk17/2(cfblk6)
  cfblk3/1 -> cfblk14/1
  cfblk1/1 -> cfblk17/3(cfblk7)
  cfblk4/2 -> cfblk8/2(cfblk8)
  cfblk10/1 -> cfblk16/Action
  cfblk10/2 -> cfblk17/Action
  cfblk18/1 -> cfblk17/1(cfblk1)
  cfblk19/1 -> cfblk16/3(cfblk12)
  cfblk5/1 -> cfblk20/1
  cfblk20/1 -> cfblk16/1(cfblk1)

== system sampleModel106/cfblk78/cfblk12/cfblk5 ==
  cfblk1 : Inport
  cfblk11 : Inport  Port=2
  cfblk10 : If  IfExpression=u1 >= 0  SampleTime=1
  cfblk14 : Subsystem  TreatAsAtomicUnit=on
  cfblk15 : Subsystem  TreatAsAtomicUnit=on
  cfblk{16..20} (5 alike) : Delay
  cfblk3 : Signum
  cfblk4 : Subsystem
  cfblk5 : Subsystem
  cfblk6 : Subsystem
  cfblk7 : Subsystem
  cfblk8 : Subsystem
  cfblk9 : Subsystem
  cfblk2 : Outport
  cfblk12 : Outport  Port=2
  cfblk13 : Outport  Port=3
  wires:
  cfblk1/1 -> cfblk3/1, cfblk8/3(cfblk9)
  cfblk15/1(cfblk2) -> cfblk5/1(cfblk1)
  cfblk14/1(cfblk2) -> cfblk2/1
  cfblk3/1 -> cfblk8/1(cfblk1), cfblk15/3(cfblk14)
  cfblk11/1 -> cfblk14/1(cfblk1), cfblk15/2(cfblk13), cfblk5/3(cfblk8)
  cfblk9/1(cfblk2) -> cfblk12/1
  cfblk8/1(cfblk2) -> cfblk6/1(cfblk1)
  cfblk8/2(cfblk10) -> cfblk4/1(cfblk1), cfblk5/4(cfblk9)
  cfblk9/2(cfblk12) -> cfblk15/1(cfblk1)
  cfblk7/1(cfblk2) -> cfblk9/2(cfblk11)
  cfblk14/3(cfblk10) -> cfblk13/1, cfblk17/1
  cfblk4/1(cfblk2) -> cfblk7/1(cfblk1)
  cfblk15/2(cfblk15) -> cfblk14/2(cfblk8)
  cfblk6/1(cfblk2) -> cfblk4/2(cfblk17)
  cfblk6/2(cfblk14) -> cfblk5/2(cfblk7)
  cfblk5/1(cfblk2) -> cfblk18/1, cfblk19/1
  cfblk6/3(cfblk15) -> cfblk7/2(cfblk11)
  cfblk10/1 -> cfblk14/Action
  cfblk10/2 -> cfblk15/Action
  cfblk14/2(cfblk9) -> cfblk16/1
  cfblk16/1 -> cfblk9/1(cfblk1)
  cfblk17/1 -> cfblk8/2(cfblk8)
  cfblk18/1 -> cfblk10/1
  cfblk19/1 -> cfblk6/3(cfblk13)
  cfblk7/2(cfblk12) -> cfblk20/1
  cfblk20/1 -> cfblk6/2(cfblk12)

== system sampleModel106/cfblk79/cfblk6/cfblk8 ==
  cfblk1 : Inport
  cfblk7 : Inport  Port=2
  cfblk8 : Inport  Port=3
  cfblk3 : simulink/Discrete/Transfer Fcn Real Zero  ZeroZ=0.75  ICPrevInput=0.0  DoSatur=off
      settings: SourceProductBaseCode=SL
  cfblk4 : Gain  Gain=[39461161.614589]
  cfblk5 : Assignment  DiagnosticForDimensions=Warning  IndexOptions=Index vector (dialog)  Indices=1  OutputSizes=1
  cfblk6 : Subsystem
  cfblk2 : Outport
  cfblk9 : Outport  Port=2
  wires:
  cfblk6/1(cfblk2) -> cfblk9/1
  cfblk1/1 -> cfblk2/1, cfblk5/1
  cfblk5/1 -> cfblk3/1
  cfblk7/1 -> cfblk6/1(cfblk1), cfblk5/2
  cfblk4/1 -> cfblk6/2(cfblk9)
  cfblk3/1 -> cfblk4/1
  cfblk8/1 -> cfblk6/3(cfblk10)
